simulink model "model2"  (R2013b)
settings: Solver=ode45  StartTime=0.0  StopTime=10.0  RelTol=1e-3
values from neighbouring files (symbols this model uses):
  A = A-B*K    [variables.m]
  B = B    [variables.m]
  C = C    [variables.m]
  K = acker(A, B, K_poles)    [variables.m]
  L = acker(A', C', L_poles)    [variables.m]
  nbar = rscale(A, B, C, D, K)    [variables.m]
libraries: simulink x1
settings Model: Creator=Sander  LastModifiedBy=Sander

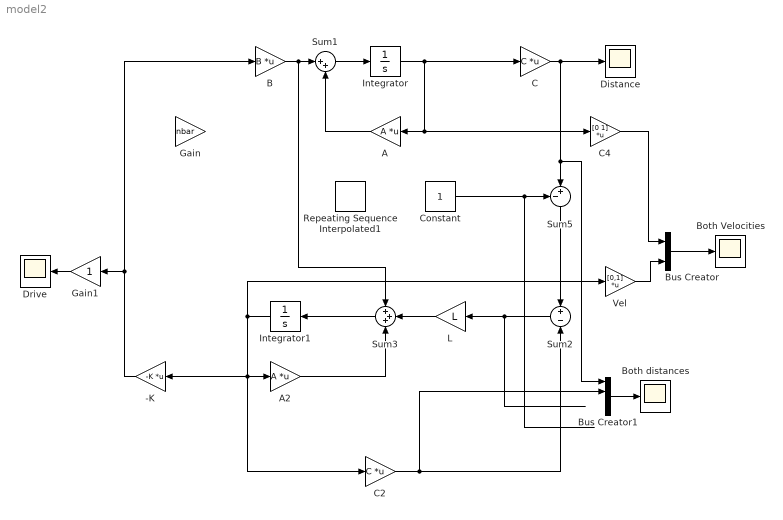
== system model2 ==
  -K : Gain  Gain=-K  Multiplication=Matrix(K*u)
  A : Gain  Gain=A  Multiplication=Matrix(K*u)
  A2 : Gain  Gain=A  Multiplication=Matrix(K*u)
  B : Gain  Gain=B  Multiplication=Matrix(K*u)
  Both Velocities : Scope
      settings: TimeRange=10  YMin=-1  YMax=1  SaveName=ScopeData2
  Both distances : Scope
      settings: TimeRange=10  YMin=-10  YMax=4  SaveName=ScopeData3
  Bus Creator : BusCreator  Inputs=2
  Bus Creator1 : BusCreator
  C : Gain  Gain=C  Multiplication=Matrix(K*u)
  C2 : Gain  Gain=C  Multiplication=Matrix(K*u)
  C4 : Gain  Gain=[0 1]  Multiplication=Matrix(K*u)
  Constant : Constant
  Distance : Scope
      settings: TimeRange=10  YMin=2.2872  YMax=2.2886
  Drive : Scope
      settings: TimeRange=10  YMin=-1e+61  YMax=0
  Gain : Gain  Gain=nbar
  Gain1 : Gain
  Integrator : Integrator  InitialCondition=[3;0]
  Integrator1 : Integrator  InitialCondition=[0;0]
  L : Gain  Gain=L
  Repeating Sequence Interpolated1 : simulink/Sources/Repeating Sequence Interpolated  OutValues=[0 0.3 0.1 0.4 0.2 0.1].'  TimeValues=[0 1 5 6 8 10].'  LookUpMeth=Interpolation-Use End Values  tsamp=0.01  OutMin=[]  OutMax=[]  OutDataTypeStr=double  OutputDataTypeScalingMode=double  OutDataType=fixdt(0,8)  OutScaling=2^-10
  Sum1 : Sum  Inputs=|++
  Sum2 : Sum  Inputs=+|-
  Sum3 : Sum  Inputs=+++
  Sum5 : Sum  Inputs=-+|
  Vel : Gain  Gain=[0,1]  Multiplication=Matrix(K*u)
  wires:
  Sum1/1 -> Integrator/1
  B/1 -> Sum3/1, Sum1/1
  Sum2/1 -> L/1
  Sum3/1 -> Integrator1/1
  A2/1 -> Sum3/3
  Integrator/1 -> C4/1, A/1, C/1
  Bus Creator/1 -> Both Velocities/1
  C4/1 -> Bus Creator/1
  Vel/1 -> Bus Creator/2
  L/1 -> Sum3/2
  Bus Creator1/1 -> Both distances/1
  C/1 -> Bus Creator1/1, Sum5/2, Distance/1
  Integrator1/1 -> C2/1, A2/1, -K/1, Vel/1
  -K/1 -> B/1, Gain1/1
  A/1 -> Sum1/2
  Gain1/1 -> Drive/1
  Sum5/1 -> Sum2/1
  Constant/1 -> Sum5/1
  C2/1 -> Bus Creator1/2, Sum2/2
